simulink model "lander_sim_simple"  (R2023a)
settings: Solver=VariableStepAuto  StartTime=0.0  StopTime=10.0  RelTol=1e-3
libraries: simulink x1, simulink_extras x1
settings Model: Creator=User  LastModifiedBy=User

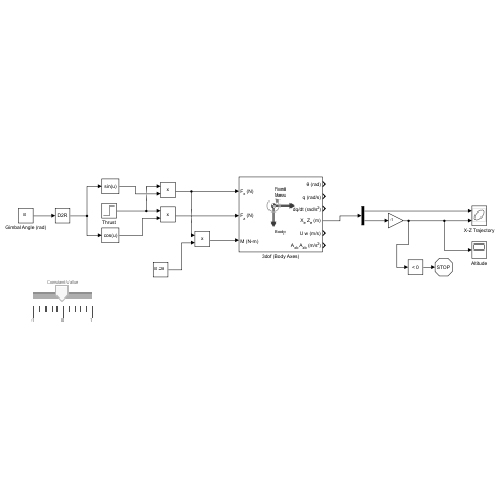
[thumbnail: Simulink's stored preview of the top-level diagram]
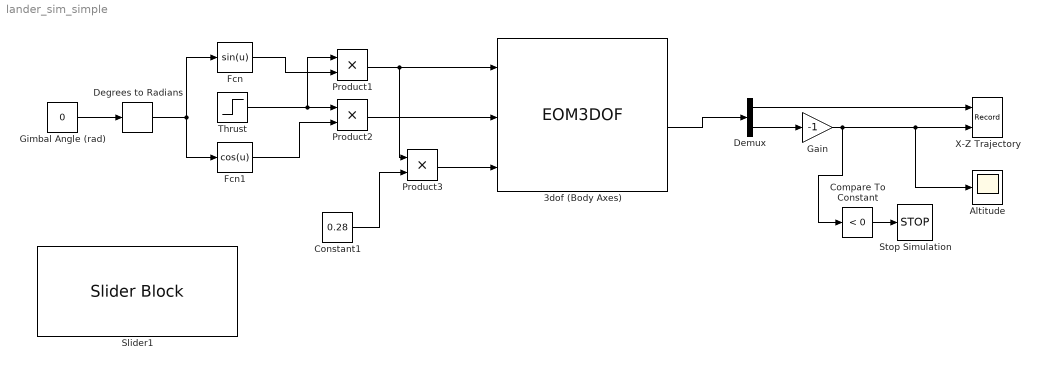
== system lander_sim_simple ==
  3dof (Body Axes) : EOM3DOF  v_ini=0  mass=0.543  Iyy=0.048
  Altitude : Scope
  Compare To Constant : simulink/Logic and Bit Operations/Compare To Constant  relop=<  const=0  OutDataTypeStr=boolean
  Constant1 : Constant  Value=0.28
  Degrees to Radians : simulink_extras/Transformations/Degrees to Radians
  Demux : Demux  Outputs=2
  Fcn : Fcn  Expr=sin(u)
  Fcn1 : Fcn  Expr=cos(u)
  Gain : Gain  Gain=-1
  Gimbal Angle (rad) : Constant  Value=0
  Product1 : Product
  Product2 : Product
  Product3 : Product
  Slider1 : SliderBlock  ScaleMin=-1  ScaleMax=1  TickInterval=1
  Stop Simulation : Stop
  Thrust : Step  Time=2  Before=-15  After=0  SampleTime=0
  X-Z Trajectory : Record  FileSettingsInternal="{\"entries\":[{\"content\":{\"excelSettings\":{\"content\":{},\"type\":\"Streamout.ExcelSettings\"}},\"type\":\"Streamout.FileSettingStorage\",\"uuid\":\"3e6c0a8b-ec00-4a1d-9dc4-1883053d7317\"}],\"packageUris\":[\"http://schema.mathworks.com/mf0/streamout_blocks/R2020a\"],\"version\":\"1.0\"}"  Layout=[1 1]  SignalsInternal="{\"entries\":[{\"content\":{\"signals\":[{\"content\":{\"blockPath\":[\"lander_sim_simple/X-Z Trajectory\"],\"dimensions\":[1],\"domain\":\"lander_sim_simple/X-Z Trajectory\",\"lineColor\":\"#a2142f\",\"plots\":[1],\"port\":1,\"signalID\":267,\"signalName\":\"Demux:1\"},\"type\":\"RecordBlkView.Signal\",\"uuid\":\"11d24867-ee11-4af1-899d-fc05cc562b6b\"},{\"content\":{\"blockPath\":[\"lander_sim_simple/X-Z Trajectory\"],\"dimensions\":[1],\"domain\":\"lander_sim_simple/X-Z Trajectory\",\"lineColor\":\"#139fff\",\"plots\":[1],\"port\":2,\"signalID\":270,\"signalName\":\"Gain\"},\"type\":\"RecordBlkView.Signal\",\"uuid\":\"8887fe6f-eecb-48f8-9b9d-18885ac03d93\"}]},\"type\":\"RecordBlkView.InputSignals\",\"uuid\":\"19ea3877-e9c6-4b71-ba83-d44025bceb20\"}],\"packageUris\":[\"http://schema.mathworks.com/mf0/streamout_blocks/R2020a\"],\"version\":\"1.0\"}"  VisualizationBindings="{\"xyplotplugin\":{\"info\":[{\"series\":[{\"bindingParametersList\":[{\"parameter\":\"X-Axis\",\"signalID\":267,\"signalName\":\"Demux:1\"},{\"parameter\":\"Y-Axis\",\"signalID\":270,\"signalName\":\"Gain\"}],\"seriesID\":32610}],\"subplotID\":1}]}}"  CompatibilityTag=XY  st=-1
  wires:
  Demux/2 -> Gain/1
  Gain/1 -> Compare To Constant/1, Altitude/1, X-Z Trajectory/2
  Compare To Constant/1 -> Stop Simulation/1
  3dof (Body Axes)/4 -> Demux/1
  Degrees to Radians/1 -> Fcn1/1, Fcn/1
  Gimbal Angle (rad)/1 -> Degrees to Radians/1
  Fcn/1 -> Product1/2
  Thrust/1 -> Product1/1, Product2/1
  Fcn1/1 -> Product2/2
  Product2/1 -> 3dof (Body Axes)/2
  Product1/1 -> Product3/1, 3dof (Body Axes)/1
  Constant1/1 -> Product3/2
  Product3/1 -> 3dof (Body Axes)/3
  Demux/1 -> X-Z Trajectory/1
